simulink library "uavsimBlockset_LongitudinalEulerAttitudeAndSpeedController"  (Simulink 8.0)
settings: Solver=ode45  StartTime=0.0  StopTime=10.0  RelTol=1e-3
undefined symbols (not defined in the file): aircraftLibraryData, DiscIntNeverNeededParam
settings Model: Creator=mstolle  LastModifiedBy=j.bolting

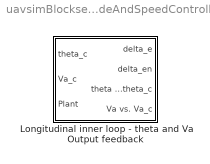
== system uavsimBlockset_LongitudinalEulerAttitudeAndSpeedController ==
  Longitudinal inner loop - theta and Va Output feedback : Subsystem  mask{mask_K=aircraftLibraryData.zagi.control.gains.Klongi_theta_Va}
      mask prompts: mask_K "Feedback gain matrix K"

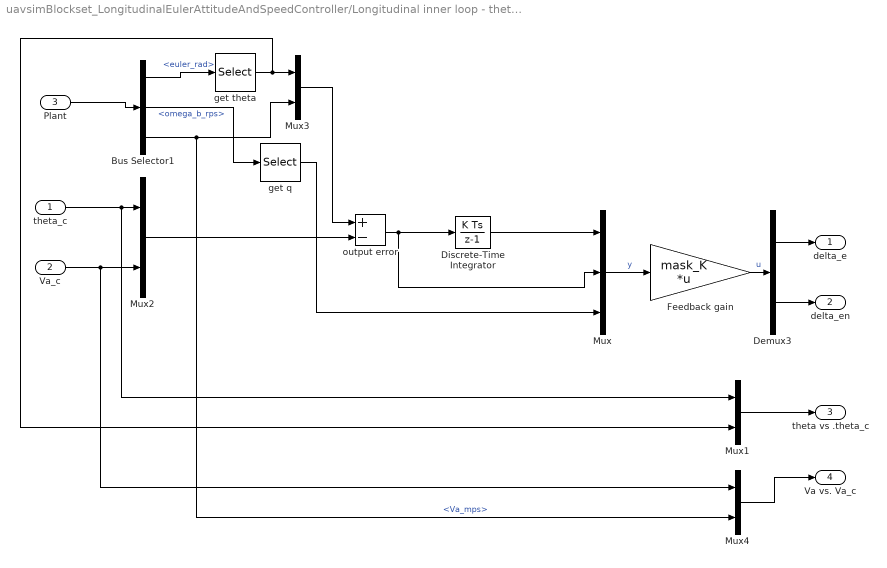
== system uavsimBlockset_LongitudinalEulerAttitudeAndSpeedController/Longitudinal inner loop - theta and Va Output feedback ==
  theta_c : Inport
  Va_c : Inport  Port=2
  Plant : Inport  Port=3  OutDataTypeStr=Bus: Airframe
  Bus Selector1 : BusSelector  OutputSignals=Kinematics.Attitude.euler_rad,Kinematics.RotationalVelocity.omega_b_rps,Aero.Va_mps
  Demux3 : Demux  Outputs=2
  Discrete-Time Integrator : DiscreteIntegrator  SampleTime=-1  ICPrevOutput=DiscIntNeverNeededParam  ICPrevScaledInput=DiscIntNeverNeededParam
  Feedback gain : Gain  Gain=mask_K  Multiplication=Matrix(K*u)
  Mux : Mux  Inputs=3
  Mux{1..4} (4 alike) : Mux  Inputs=2
  get q : Selector  InputPortWidth=3  IndexOptions=Index vector (dialog)  Indices=2  OutputSizes=1
  get theta : Selector  InputPortWidth=3  IndexOptions=Index vector (dialog)  Indices=2  OutputSizes=1
  output error : Sum  Inputs=+-
  delta_e : Outport
  delta_en : Outport  Port=2
  theta vs .theta_c : Outport  Port=3
  Va vs. Va_c : Outport  Port=4
  wires:
  Mux/1 -> Feedback gain/1  "y"
  output error/1 -> Mux/2, Discrete-Time Integrator/1
  Mux2/1 -> output error/2
  Mux3/1 -> output error/1
  theta_c/1 -> Mux1/1, Mux2/1
  Va_c/1 -> Mux4/1, Mux2/2
  Plant/1 -> Bus Selector1/1
  Feedback gain/1 -> Demux3/1  "u"
  Demux3/1 -> delta_e/1
  Demux3/2 -> delta_en/1
  Bus Selector1/2 -> get q/1  "<omega_b_rps>"
  get q/1 -> Mux/3
  Bus Selector1/3 -> Mux4/2, Mux3/2  "<Va_mps>"
  Bus Selector1/1 -> get theta/1  "<euler_rad>"
  get theta/1 -> Mux1/2, Mux3/1
  Mux1/1 -> theta vs .theta_c/1
  Mux4/1 -> Va vs. Va_c/1
  Discrete-Time Integrator/1 -> Mux/1
